simulink model "ex3_linearized"  (R2020b)
settings: Solver=ode45  StartTime=0.0  StopTime=10  MaxStep=0.5*10^-2  RelTol=1e-9
values from neighbouring files (symbols this model uses):
  C = 0.0157    [ex2_1.m]    (also in ex3.m = 3.73e-06; ex4.m = [1 0]; mp62.m = [1 0]; od.m = [1 0;0 0])
  c = 0.1    [ex1.m]    (also in ex2_1.m; ex3.m; ex4.m; od.m)
  Ib = 50E-3    (= 0.05)    [ex3.m]    (also in ex4.m; od.m)
  k = linspace(-5,5,1000)    [OP2_dynamicEstimation.m]    (also in dynamicEstimation.m = x2; ex1.m = 100; ex2_1.m = 100; ex3.m = 1272.8)
  l = dynamicEstimation(x1,y1,x2,y2,10)    [OP2_dynamicEstimation.m]    (also in ex1.m = 0.0003; ex2_1.m = 0.0003; ex3.m = 0.0003)
  m = 1    [ex1.m]    (also in ex2_1.m; ex3.m = 0.48; ex4.m = 0.48; od.m = 0.48)
libraries: pid_lib x1
settings Model: OrderedModelArguments=off  Creator=danli  LastModifiedBy=danli

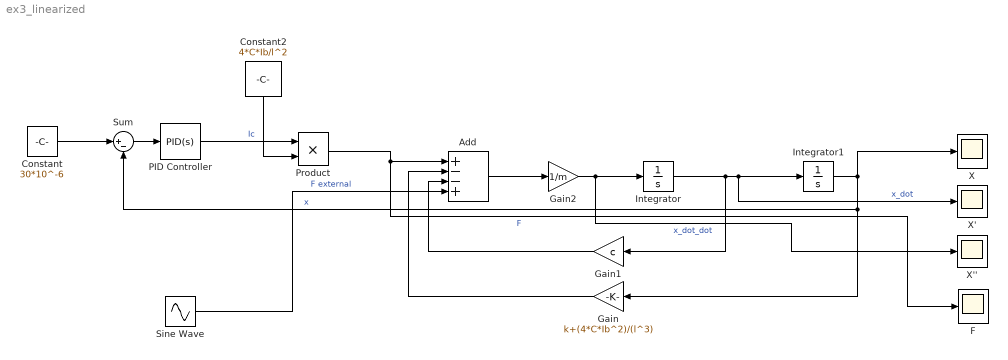
== system ex3_linearized ==
  Add : Sum  Inputs=+--+
  Constant : Constant  Value=30*10^-6
  Constant2 : Constant  Value=4*C*Ib/l^2
  F : Scope
  Gain : Gain  Gain=k+(4*C*Ib^2)/(l^3)
  Gain1 : Gain  Gain=c
  Gain2 : Gain  Gain=1/m
  Integrator : Integrator
  Integrator1 : Integrator  InitialCondition=50*10^-6
  PID Controller : pid_lib/PID Controller  Controller=PID  Form=Parallel  TimeDomain=Continuous-time  UseExternalTs=off  SampleTime=-1  IntegratorMethod=Forward Euler  FilterMethod=Forward Euler  ControllerParametersSource=internal  P=7433.33  I=2500  D=8.1549  UseFilter=on  N=100  TunerSelectOption=Frequency Response Based  InitialConditionSource=internal  InitialConditionForIntegrator=0  InitialConditionForFilter=0  DifferentiatorICPrevScaledInput=0  ExternalReset=none  TrackingMode=off  Kt=1  LimitOutput=off  SatLimitsSource=internal  UpperSaturationLimit=inf  LowerSaturationLimit=-inf  LinearizeAsGain=on  AntiWindupMode=none  Kb=1  POutMin=[]  POutMax=[]  IOutMin=[]  IOutMax=[]  DOutMin=[]  DOutMax=[]  NOutMin=[]  NOutMax=[]  SumOutMin=[]  SumOutMax=[]  SaturationOutMin=[]  SaturationOutMax=[]  PParamMin=[]  PParamMax=[]  IParamMin=[]  IParamMax=[]  DParamMin=[]  DParamMax=[]  NParamMin=[]  NParamMax=[]  KbParamMin=[]  KbParamMax=[]  KtParamMin=[]  KtParamMax=[]  KbOutMin=[]  KbOutMax=[]  KtOutMin=[]  KtOutMax=[]  IntegratorOutMin=[]  IntegratorOutMax=[]  FilterOutMin=[]  FilterOutMax=[]  SumI1OutMin=[]  SumI1OutMax=[]  SumI2OutMin=[]  SumI2OutMax=[]  SumI3OutMin=[]  SumI3OutMax=[]  SumI4OutMin=[]  SumI4OutMax=[]  SumDOutMin=[]  SumDOutMax=[]  DifferentiatorOutMin=[]  DifferentiatorOutMax=[]  FilterDiffOutCoefMin=[]  FilterDiffOutCoefMax=[]  ReciprocalOutMin=[]  ReciprocalOutMax=[]  SumDenOutMin=[]  SumDenOutMax=[]  SumNumOutMin=[]  SumNumOutMax=[]  DivideOutMin=[]  DivideOutMax=[]  UdiffTsProdOutMin=[]  UdiffTsProdOutMax=[]  NTsProdOutMin=[]  NTsProdOutMax=[]  UintegralTsProdOutMin=[]  UintegralTsProdOutMax=[]  UngainTsProdOutMin=[]  UngainTsProdOutMax=[]  IntegratorContinuousStateAttributes=''  IntegratorStateMustResolveToSignalObject=off  IntegratorRTWStateStorageClass=Auto  FilterContinuousStateAttributes=''  FilterStateMustResolveToSignalObject=off  FilterRTWStateStorageClass=Auto  ParallelPVariant=InternalParameters  IdealPVariant=Disabled  IVariant=InternalParameters  DVariant=InternalParameters  IntegratorVariant=Continuous  SatVariant=Disabled  AWVariant=Passthrough  PCopyVariant=Disabled  TRVariant=Disabled  FdbkBlocksVariant=Forward  IdealPFdbkVariant=Disabled  SatFdbkVariant=Disabled  DerivativeFilterVariant=ContFilter  NVariant=InternalParameters  NCopyVariant=Disabled  FilterICVariant=InternalICsFilter  IntegratorICVariant=InternalICs  ExternalResetVariant=Disabled  TRSumVariant=Passthrough  SumFdbkVariant=Disabled  SumVariant=Sum_PID  TsampFilterVariant=InternalTs  TsampNgainVariant=Passthrough  TsampIntegralVariant=Passthrough  ExternalSaturationOutDataTypeStr=Inherit: Same as second input
  Product : Product  Inputs=**
  Sine Wave : Sin  Amplitude=13  Frequency=230  SampleTime=0
  Sum : Sum  Inputs=|+-
  X : Scope
  X' : Scope
  X'' : Scope
  wires:
  Constant/1 -> Sum/1
  Sum/1 -> PID Controller/1
  PID Controller/1 -> Product/1  "Ic"
  Sine Wave/1 -> Add/4  "F external"
  Integrator1/1 -> Sum/2, Gain/1, X/1  "x"
  Gain1/1 -> Add/3
  Integrator/1 -> X'/1, Integrator1/1, Gain1/1  "x_dot"
  Gain/1 -> Add/2
  Add/1 -> Gain2/1
  Product/1 -> F/1, Add/1  "F"
  Constant2/1 -> Product/2
  Gain2/1 -> X''/1, Integrator/1  "x_dot_dot"
